simulink model "radia_maglev"  (R2026a)
settings: Solver=FixedStepDiscrete  StopTime=0.1  FixedStep=0.0001
model workspace (MAT data in the model file):
  radia_maglev_current_amplitude_A = 20
  radia_maglev_family.schema = "radia.hcurl.eddy_foster.family.v1"
  radia_maglev_family.source_file = ""
  radia_maglev_family.shared_modes = 1
  radia_maglev_family.positions_m = [0; 0.01]
  radia_maglev_family.decay_rates = [160; 950]
  radia_maglev_family.modal_port_rhs = reshape([0.3 0.12 0.24 0.1], [2 1 2])
  radia_maglev_family.force_operator = reshape([0 0 -0.18 0 0 -0.08 0 0 -0.135 0 0 -0.06], [3 2 1 2])
  radia_maglev_family.Ad = [0.984127320055  0; 0  0.909372934468]
  radia_maglev_family.bd_gain = [9.92042496545e-05; 9.53969110861e-05]
  radia_maglev_family.x0 = [0; 0]
  radia_maglev_family.snapshot_count = 2
  radia_maglev_family.state_order = 2
  radia_maglev_family.port_count = 1
  radia_maglev_family.sample_time_s = 0.0001
  radia_maglev_family.interpolation = "linear"
  radia_maglev_family.extrapolation = "error"
  radia_maglev_family.metadata.purpose = "diagnostic-smoke-only"
  radia_maglev_family.metadata.production_replacement = "radia.vim.ExportHCurlEddyFosterFamilyJSON"
  radia_maglev_frequency_Hz = 50
settings Model: Creator=Administrator  LastModifiedBy=Administrator

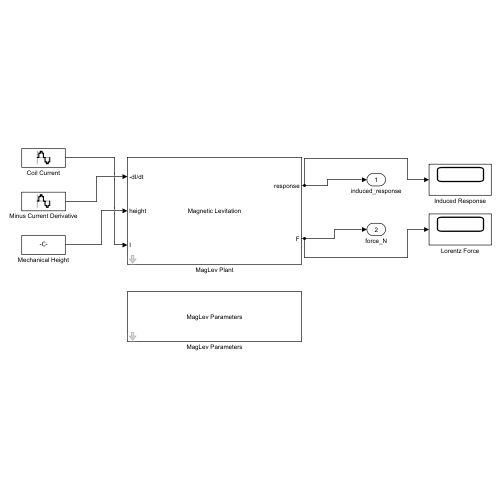
[thumbnail: Simulink's stored preview of the top-level diagram]
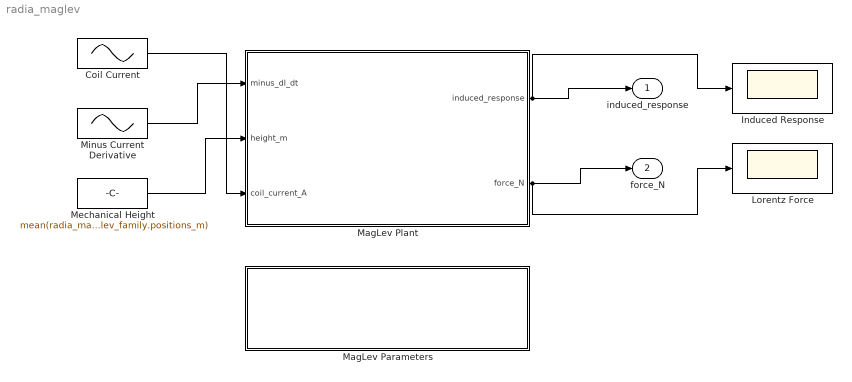
== system radia_maglev ==
  Coil Current : Sin  Amplitude=radia_maglev_current_amplitude_A  Frequency=2*pi*radia_maglev_frequency_Hz  SampleTime=radia_maglev_family.sample_time_s
  Induced Response : Scope
  Lorentz Force : Scope
  MagLev Parameters : Subsystem  mask{family_file=, interpolation=linear, extrapolation=error, sample_time_s=0.0001}
      mask prompts: family_file "Foster family JSON"; interpolation "Position interpolation"; extrapolation "Outside sampled range"; sample_time_s "Sample time (s)"
      mask help: Load a shared-mode Foster HCurl family exported by Radia. The empty path keeps the family embedded in this model.
      mask Callback family_file: radia.simulink.onMagLevFamilyChanged(gcb);
      mask TypeOptions interpolation: nearest | linear | pchip
      mask Callback interpolation: radia.simulink.onMagLevFamilyChanged(gcb);
      mask TypeOptions extrapolation: error | clamp
      mask Callback extrapolation: radia.simulink.onMagLevFamilyChanged(gcb);
      mask Callback sample_time_s: radia.simulink.onMagLevFamilyChanged(gcb);
      mask Display: disp('MagLev Parameters');
  MagLev Plant : Subsystem  Tag=RadiaMagLevFoster  mask{family=radia_maglev_family}
      mask prompts: family "Shared-mode Foster family"
      mask help: Moving conductive-body HCurl plant in Foster modal form. One mode set is shared by every height; the block evaluates the induced response and reduced Lorentz force without per-step Python.
      mask Callback family: radia.simulink.onMagLevBlockFamilyChanged(gcb);
      mask Display: disp('Magnetic Levitation');port_label('input',1,'-dI/dt');port_label('input',2,'height');port_label('input',3,'I');port_label('output',1,'response');port_label('output',2,'F');
  Mechanical Height : Constant  Value=mean(radia_maglev_family.positions_m)
  Minus Current Derivative : Sin  Amplitude=2*pi*radia_maglev_frequency_Hz*radia_maglev_current_amplitude_A  Frequency=2*pi*radia_maglev_frequency_Hz  Phase=-pi/2  SampleTime=radia_maglev_family.sample_time_s
  induced_response : Outport
  force_N : Outport  Port=2
  wires:
  Minus Current Derivative/1 -> MagLev Plant/1(minus_dI_dt)
  Mechanical Height/1 -> MagLev Plant/2(height_m)
  Coil Current/1 -> MagLev Plant/3(coil_current_A)
  MagLev Plant/1(induced_response) -> induced_response/1, Induced Response/1
  MagLev Plant/2(force_N) -> force_N/1, Lorentz Force/1

== system radia_maglev/MagLev Parameters ==

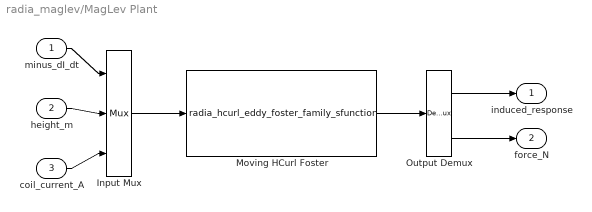
== system radia_maglev/MagLev Plant ==
  minus_dI_dt : Inport
  height_m : Inport  Port=2
  coil_current_A : Inport  Port=3
  Input Mux : Mux  Inputs=3
  Moving HCurl Foster : M-S-Function  FunctionName=radia_hcurl_eddy_foster_family_sfunction  Parameters=radia_maglev_family
  Output Demux : Demux  Outputs=[-1 3]
  induced_response : Outport
  force_N : Outport  Port=2
  wires:
  minus_dI_dt/1 -> Input Mux/1
  height_m/1 -> Input Mux/2
  coil_current_A/1 -> Input Mux/3
  Input Mux/1 -> Moving HCurl Foster/1
  Moving HCurl Foster/1 -> Output Demux/1
  Output Demux/1 -> induced_response/1
  Output Demux/2 -> force_N/1
